simulink model "SimuModel_J_adaptive"  (Simulink 9.3)
settings: Solver=ode23  StartTime=0.0  StopTime=t_d  MaxStep=Tc  RelTol=1e-8  AbsTol=1e-8
values from neighbouring files (symbols this model uses):
  F_v = K_r*diag([0.01 0.01])*K_r    [InitVariable_exe.m]
  g = 9.81    [InitVariable_exe.m]
  K_d = 750*diag([1 1])    [InitVariable_exe.m]
  K_ml = 0.01    [InitVariable_exe.m]
  Lam = 5*diag([1 1])    [InitVariable_exe.m]
  m_l0 = 0    [InitVariable_exe.m]
  q_i = [-1.4706; 2.9413]    [InitVariable_exe.m]
  Tc = 0.001    [InitVariable_exe.m]
  Ts = Tc    (= 0.001)    [InitVariable_exe.m]
undefined symbols (not defined in the file or in its folder): a, BMatrix, DiscIntNeverNeededParam, pi_l
settings Model: Creator=luigivillani  LastModifiedBy=yuzg  ExtModeAutoUpdateStatusClock=off
settings SolverCC: AutoScaleAbsTol=off  InitialStep=0.1*Tc
settings DataIOCC: SaveOutput=off  SaveTime=off
settings OptimizationCC: BlockReduction=off  BooleanDataType=off  ExpressionDepthLimit=2147483647  InitFltsAndDblsToZero=on
settings DebuggingCC: SaveWithParameterizedLinksMsg=none  SignalResolutionControl=TryResolveAllWithWarning  MultiTaskDSMMsg=warning  MultiTaskCondExecSysMsg=none  StateNameClashWarn=warning
settings HardwareCC: TargetUnknown=on
settings SFSimCC: SimUseLocalCustomCode=on
settings RTWCC: RTWUseLocalCustomCode=on
settings GRTTargetCC: TargetFcnLib=ansi_tfl_tmw.mat
settings ConfigComp: CovExternalEMLEnable=on

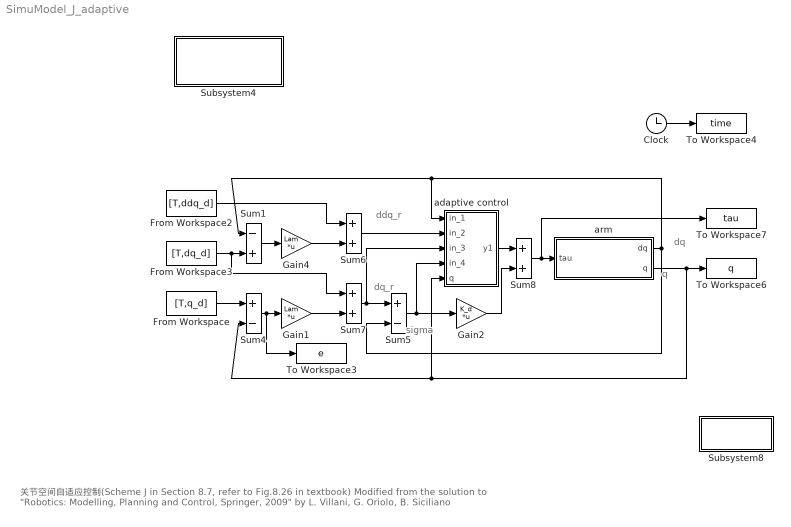
== system SimuModel_J_adaptive ==
  note: sigma
  note: dq_r
  note: ddq_r
  note: dq
  note: q
  note: 关节空间自适应控制(Scheme J in Section 8.7, refer to Fig.8.26 in textbook)
      | Modified from the solution to "Robotics: Modelling, Planning and Control, Springer, 2009" by L. Villani, G. Oriolo, B. Siciliano
  Clock : Clock
  From Workspace : FromWorkspace  VariableName=[T,q_d]  SampleTime=Tc
  From Workspace2 : FromWorkspace  VariableName=[T,ddq_d]  SampleTime=Tc
  From Workspace3 : FromWorkspace  VariableName=[T,dq_d]  SampleTime=Tc
  Gain1 : Gain  Gain=Lam  Multiplication=Matrix(K*u)  SampleTime=Tc
      mask Display: disp('Lam')
  Gain2 : Gain  Gain=K_d  Multiplication=Matrix(K*u)  SampleTime=Tc
      mask Display: disp('K_d')
  Gain4 : Gain  Gain=Lam  Multiplication=Matrix(K*u)  SampleTime=Tc
      mask Display: disp('Lam')
  Subsystem4 : Subsystem
      settings: OpenFcn=clear all;c=0;InitVariable_exe;
      mask Display: disp('lambda=5\nK_d = 750I\nk_pai(k_ml)=0.01')
  Subsystem8 : Subsystem
      settings: OpenFcn=PlotFigure;
      mask Display: disp('plot')
  Sum1 : Sum  Inputs=-+  SampleTime=Tc  SaturateOnIntegerOverflow=on  InputSameDT=on  OutDataTypeStr=Inherit: Same as first input
  Sum4 : Sum  Inputs=+-  SampleTime=Tc  SaturateOnIntegerOverflow=on  InputSameDT=on  OutDataTypeStr=Inherit: Same as first input
  Sum5 : Sum  Inputs=+-  SampleTime=Tc  SaturateOnIntegerOverflow=on  InputSameDT=on  OutDataTypeStr=Inherit: Same as first input
  Sum6 : Sum  SaturateOnIntegerOverflow=on  InputSameDT=on  OutDataTypeStr=Inherit: Same as first input
  Sum7 : Sum  SaturateOnIntegerOverflow=on  InputSameDT=on  OutDataTypeStr=Inherit: Same as first input
  Sum8 : Sum  SaturateOnIntegerOverflow=on  InputSameDT=on  OutDataTypeStr=Inherit: Same as first input
  To Workspace3 : ToWorkspace  VariableName=e  SampleTime=Ts
      settings: MaxDataPoints=5001
  To Workspace4 : ToWorkspace  VariableName=time  SampleTime=Ts
      settings: MaxDataPoints=5001
  To Workspace6 : ToWorkspace  VariableName=q  SampleTime=Ts
      settings: MaxDataPoints=5001
  To Workspace7 : ToWorkspace  VariableName=tau  SampleTime=Ts
      settings: MaxDataPoints=5001
  adaptive control : Subsystem
      mask Display: disp('Y( . )pi_h')
  arm : Subsystem
      mask Display: disp('Robot InvDynamics')
  wires:
  Clock/1 -> To Workspace4/1
  Sum1/1 -> Gain4/1
  From Workspace/1 -> Sum4/1
  Sum4/1 -> To Workspace3/1, Gain1/1
  Gain1/1 -> Sum7/2
  Sum6/1 -> adaptive control/2(in_2)
  Sum8/1 -> To Workspace7/1, arm/1(tau)
  adaptive control/1(y1) -> Sum8/1
  Sum5/1 -> adaptive control/4(in_4), Gain2/1
  Gain2/1 -> Sum8/2
  Gain4/1 -> Sum6/2
  From Workspace2/1 -> Sum6/1
  From Workspace3/1 -> Sum1/2, Sum7/1
  Sum7/1 -> Sum5/1, adaptive control/3(in_3)
  arm/2("q ") -> To Workspace6/1, Sum4/2, adaptive control/5(q)
  arm/1(dq) -> adaptive control/1(in_1), Sum1/1, Sum5/2

== system SimuModel_J_adaptive/Subsystem4 ==
  note: start

== system SimuModel_J_adaptive/Subsystem8 ==
  note: start

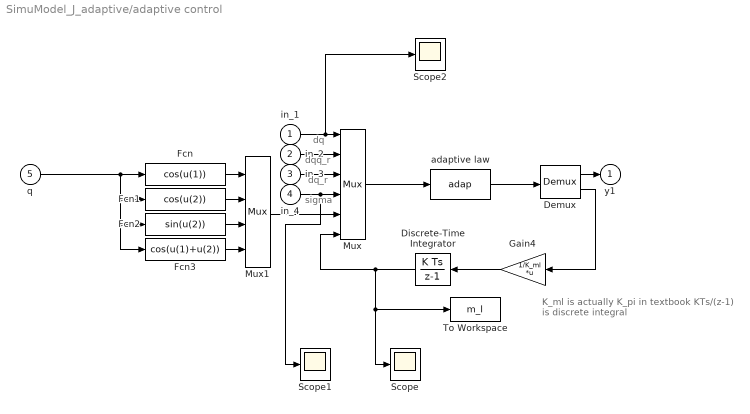
== system SimuModel_J_adaptive/adaptive control ==
  note: K_ml is actually K_pi in textbook
      | KTs/(z-1) is discrete integral
  note: dq
  note: dqq_r
  note: dq_r
  note: sigma
  in_1 : Inport
  in_2 : Inport  Port=2
  in_3 : Inport  Port=3
  in_4 : Inport  Port=4
  q : Inport  Port=5
  Demux : Demux  Outputs=[2;1]
  Discrete-Time Integrator : DiscreteIntegrator  InitialCondition=m_l0  SampleTime=Tc  ICPrevOutput=DiscIntNeverNeededParam  ICPrevScaledInput=DiscIntNeverNeededParam
  Fcn : Fcn  Expr=cos(u(1))  SampleTime=Tc
  Fcn1 : Fcn  Expr=cos(u(2))  SampleTime=Tc
  Fcn2 : Fcn  Expr=sin(u(2))  SampleTime=Tc
  Fcn3 : Fcn  Expr=cos(u(1)+u(2))  SampleTime=Tc
  Gain4 : Gain  Gain=1/K_ml  Multiplication=Matrix(K*u)  SampleTime=Tc
      mask Display: disp('1/K_ml')
  Mux : Mux  Inputs=[2;2;2;2;4;1]
  Mux1 : Mux
  Scope : Scope
  Scope1 : Scope
  Scope2 : Scope
  To Workspace : ToWorkspace  VariableName=m_l  SampleTime=Ts
      settings: MaxDataPoints=5001
  adaptive law : MATLABFcn  MATLABFcn=adap  OutputDimensions=3  SampleTime=Tc
      mask Display: disp('adap')
  y1 : Outport  InitialOutput=0
  wires:
  in_4/1 -> Scope1/1, Mux/4
  Mux1/1 -> Mux/5
  Fcn3/1 -> Mux1/4
  Fcn2/1 -> Mux1/3
  Fcn1/1 -> Mux1/2
  Fcn/1 -> Mux1/1
  in_3/1 -> Mux/3
  in_2/1 -> Mux/2
  adaptive law/1 -> Demux/1
  Demux/1 -> y1/1
  Gain4/1 -> Discrete-Time Integrator/1
  Demux/2 -> Gain4/1
  in_1/1 -> Scope2/1, Mux/1
  Mux/1 -> adaptive law/1
  q/1 -> Fcn/1, Fcn1/1, Fcn2/1, Fcn3/1
  Discrete-Time Integrator/1 -> Scope/1, To Workspace/1, Mux/6

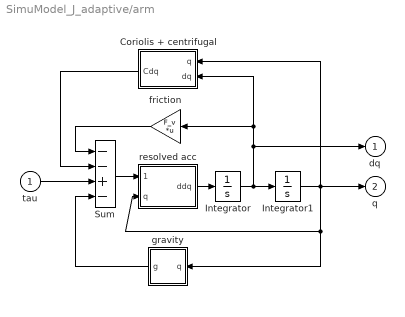
== system SimuModel_J_adaptive/arm ==
  tau : Inport
  Coriolis + centrifugal : Subsystem
      mask Display: disp('C(q,dq)dq')
  Integrator : Integrator  InitialCondition=[0 0]  ZeroCross=off
  Integrator1 : Integrator  InitialCondition=q_i  ZeroCross=off
  Sum : Sum  Inputs=--+-  SaturateOnIntegerOverflow=on  InputSameDT=on  OutDataTypeStr=Inherit: Same as first input
  friction : Gain  Gain=F_v  Multiplication=Matrix(K*u)  SaturateOnIntegerOverflow=on  OutDataTypeStr=Inherit: Same as input  ParamDataTypeStr=Inherit: Same as input
      mask Display: disp('F_v')
  gravity : Subsystem
      mask Display: disp('g(q)')
  resolved acc : Subsystem
      mask Display: disp('inv(B(q))')
  dq : Outport  InitialOutput=0
  "q " : Outport  Port=2  InitialOutput=0
  wires:
  Coriolis + centrifugal/1(Cdq) -> Sum/2
  tau/1 -> Sum/3
  Integrator1/1 -> Coriolis + centrifugal/1(q), resolved acc/2(q), gravity/1(q), "q "/1
  resolved acc/1(ddq) -> Integrator/1
  Integrator/1 -> Integrator1/1, dq/1, Coriolis + centrifugal/2(dq), friction/1
  Sum/1 -> resolved acc/1(tau-tau')
  friction/1 -> Sum/1
  gravity/1(g) -> Sum/4

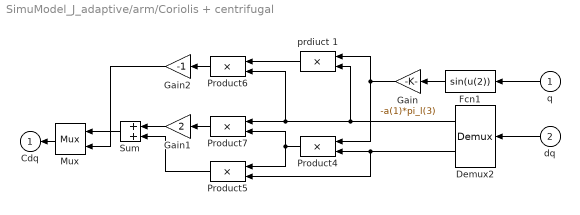
== system SimuModel_J_adaptive/arm/Coriolis + centrifugal ==
  q : Inport
  dq : Inport  Port=2
  Demux2 : Demux  Outputs=2
  Fcn1 : Fcn  Expr=sin(u(2))
  Gain : Gain  Gain=-a(1)*pi_l(3)  SaturateOnIntegerOverflow=on  OutDataTypeStr=Inherit: Same as input  ParamDataTypeStr=Inherit: Same as input
      mask Display: disp('k_3')
  Gain1 : Gain  Gain=2  SaturateOnIntegerOverflow=on  OutDataTypeStr=Inherit: Same as input  ParamDataTypeStr=Inherit: Same as input
  Gain2 : Gain  Gain=-1  SaturateOnIntegerOverflow=on  OutDataTypeStr=Inherit: Same as input  ParamDataTypeStr=Inherit: Same as input
  Mux : Mux  Inputs=2
  Product{4..7} (4 alike) : Product  SaturateOnIntegerOverflow=on  RndMeth=Zero  InputSameDT=on  OutDataTypeStr=Inherit: Same as first input
  Sum : Sum  SaturateOnIntegerOverflow=on  InputSameDT=on  OutDataTypeStr=Inherit: Same as first input
  prdiuct 1 : Product  SaturateOnIntegerOverflow=on  RndMeth=Zero  InputSameDT=on  OutDataTypeStr=Inherit: Same as first input
  Cdq : Outport  InitialOutput=0
  wires:
  dq/1 -> Demux2/1
  Gain2/1 -> Mux/2
  Product6/1 -> Gain2/1
  Mux/1 -> Cdq/1
  Sum/1 -> Mux/1
  Product5/1 -> Sum/2
  Gain1/1 -> Sum/1
  Product7/1 -> Gain1/1
  Demux2/1 -> prdiuct 1/2, Product6/2, Product7/1
  Demux2/2 -> Product4/2, Product5/2
  prdiuct 1/1 -> Product6/1
  Gain/1 -> prdiuct 1/1, Product4/1
  Fcn1/1 -> Gain/1
  q/1 -> Fcn1/1
  Product4/1 -> Product5/1, Product7/2

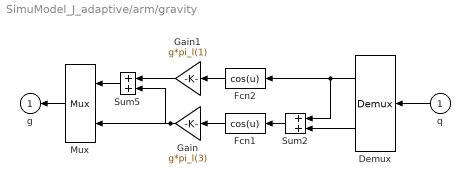
== system SimuModel_J_adaptive/arm/gravity ==
  q : Inport
  Demux : Demux  Outputs=2
  Fcn1 : Fcn  Expr=cos(u)
  Fcn2 : Fcn  Expr=cos(u)
  Gain : Gain  Gain=g*pi_l(3)  SaturateOnIntegerOverflow=on  OutDataTypeStr=Inherit: Same as input  ParamDataTypeStr=Inherit: Same as input
      mask Display: disp('k_2')
  Gain1 : Gain  Gain=g*pi_l(1)  SaturateOnIntegerOverflow=on  OutDataTypeStr=Inherit: Same as input  ParamDataTypeStr=Inherit: Same as input
      mask Display: disp('k_1')
  Mux : Mux  Inputs=2
  Sum2 : Sum  SaturateOnIntegerOverflow=on  InputSameDT=on  OutDataTypeStr=Inherit: Same as first input
  Sum5 : Sum  SaturateOnIntegerOverflow=on  InputSameDT=on  OutDataTypeStr=Inherit: Same as first input
  g : Outport  InitialOutput=0
  wires:
  q/1 -> Demux/1
  Demux/2 -> Sum2/2
  Sum2/1 -> Fcn1/1
  Fcn1/1 -> Gain/1
  Fcn2/1 -> Gain1/1
  Demux/1 -> Fcn2/1, Sum2/1
  Gain1/1 -> Sum5/1
  Sum5/1 -> Mux/1
  Gain/1 -> Sum5/2, Mux/2
  Mux/1 -> g/1

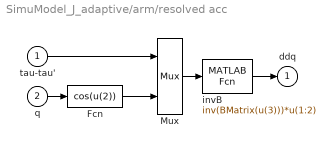
== system SimuModel_J_adaptive/arm/resolved acc ==
  tau-tau' : Inport
  q : Inport  Port=2
  Fcn : Fcn  Expr=cos(u(2))
  Mux : Mux  Inputs=[2,1]
  "invB " : MATLABFcn  MATLABFcn=inv(BMatrix(u(3)))*u(1:2)  OutputDimensions=2
      mask Display: disp('inv(B(q))')
  ddq : Outport  InitialOutput=0
  wires:
  Fcn/1 -> Mux/2
  q/1 -> Fcn/1
  "invB "/1 -> ddq/1
  tau-tau'/1 -> Mux/1
  Mux/1 -> "invB "/1
